simulink library "libMdl_normQuat"  (R2018a)
settings: Solver=VariableStepAuto  StartTime=0.0  StopTime=10.0  RelTol=1e-3
settings Model: Creator=hwinter  LastModifiedBy=Hanno

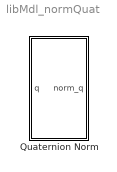
== system libMdl_normQuat ==
  Quaternion Norm : Subsystem
      mask Display:
      | color('black')
      | port_label('input',1,'q')
      | port_label('output',1,'|q|')

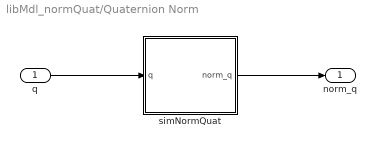
== system libMdl_normQuat/Quaternion Norm ==
  q : Inport
  simNormQuat : MATLAB Function  TreatAsAtomicUnit=on
  norm_q : Outport
  wires:
  q/1 -> simNormQuat/1(q)
  simNormQuat/1(norm_q) -> norm_q/1

== matlab function libMdl_normQuat/Quaternion Norm/simNormQuat ==
  data: q input; norm_q output
function norm_q = simNormQuat(q)

norm_q = normQuat(q);

end % function
